simulink model "IEEE_13_BUS_Radial"  (R2021b)
settings: Solver=VariableStepAuto  StartTime=0.0  StopTime=48  RelTol=1e-3
undefined symbols (not defined in the file or in its folder): f611, f632, f633, f634, f645, f646, f650, f652, f671, f675, f680, f684, f692
libraries: simulink x416, slpidlib x13
(part 6 of 7)

== system IEEE_13_BUS_Radial/f645/CONTROLLERS/lPoLC15 ==
  Sum : Sum  Inputs=|++
  base : simulink/Sources/Repeating Sequence Stair  OutValues=f645.PoLC15.l  tsamp=f645.PoLC15.ST  OutMin=[]  OutMax=[]  OutDataTypeStr=double  OutputDataTypeScalingMode=double  OutDataType=fixdt(0,8)  ConRadixGroup=Best Precision: Vector-wise  OutScaling=2^-12
  noise : simulink/Sources/Band-Limited White Noise  Cov=f645.PoLC15.Noise  Ts=f645.PoLC15.NoiseST  seed=f645.PoLC15.NoiseSD
  P : Outport  VectorParamsAs1DForOutWhenUnconnected=off
  wires:
  Sum/1 -> P/1
  noise/1 -> Sum/2
  base/1 -> Sum/1

== system IEEE_13_BUS_Radial/f645/CONTROLLERS/lPoLC16 ==
  cv : Inport
  Sum : Sum  Inputs=|++
  Terminator : Terminator
  base : simulink/Sources/Repeating Sequence Stair  OutValues=f645.PoLC16.l  tsamp=f645.PoLC16.ST  OutMin=[]  OutMax=[]  OutDataTypeStr=double  OutputDataTypeScalingMode=double  OutDataType=fixdt(0,8)  ConRadixGroup=Best Precision: Vector-wise  OutScaling=2^-12
  noise : simulink/Sources/Band-Limited White Noise  Cov=f645.PoLC16.Noise  Ts=f645.PoLC16.NoiseST  seed=f645.PoLC16.NoiseSD
  P : Outport  VectorParamsAs1DForOutWhenUnconnected=off
  wires:
  Sum/1 -> Terminator/1
  noise/1 -> Sum/2
  base/1 -> Sum/1
  cv/1 -> P/1

== system IEEE_13_BUS_Radial/f645/CONTROLLERS/lPoLC2 ==
  Sum : Sum  Inputs=|++
  base : simulink/Sources/Repeating Sequence Stair  OutValues=f645.PoLC2.l  tsamp=f645.PoLC2.ST  OutMin=[]  OutMax=[]  OutDataTypeStr=double  OutputDataTypeScalingMode=double  OutDataType=fixdt(0,8)  ConRadixGroup=Best Precision: Vector-wise  OutScaling=2^-12
  noise : simulink/Sources/Band-Limited White Noise  Cov=f645.PoLC2.Noise  Ts=f645.PoLC2.NoiseST  seed=f645.PoLC2.NoiseSD
  P : Outport  VectorParamsAs1DForOutWhenUnconnected=off
  wires:
  Sum/1 -> P/1
  noise/1 -> Sum/2
  base/1 -> Sum/1

== system IEEE_13_BUS_Radial/f645/CONTROLLERS/lPoLC3 ==
  Sum : Sum  Inputs=|++
  base : simulink/Sources/Repeating Sequence Stair  OutValues=f645.PoLC3.l  tsamp=f645.PoLC3.ST  OutMin=[]  OutMax=[]  OutDataTypeStr=double  OutputDataTypeScalingMode=double  OutDataType=fixdt(0,8)  ConRadixGroup=Best Precision: Vector-wise  OutScaling=2^-12
  noise : simulink/Sources/Band-Limited White Noise  Cov=f645.PoLC3.Noise  Ts=f645.PoLC3.NoiseST  seed=f645.PoLC3.NoiseSD
  P : Outport  VectorParamsAs1DForOutWhenUnconnected=off
  wires:
  Sum/1 -> P/1
  noise/1 -> Sum/2
  base/1 -> Sum/1

== system IEEE_13_BUS_Radial/f645/CONTROLLERS/lPoLC4 ==
  Sum : Sum  Inputs=|++
  base : simulink/Sources/Repeating Sequence Stair  OutValues=f645.PoLC4.l  tsamp=f645.PoLC4.ST  OutMin=[]  OutMax=[]  OutDataTypeStr=double  OutputDataTypeScalingMode=double  OutDataType=fixdt(0,8)  ConRadixGroup=Best Precision: Vector-wise  OutScaling=2^-12
  noise : simulink/Sources/Band-Limited White Noise  Cov=f645.PoLC4.Noise  Ts=f645.PoLC4.NoiseST  seed=f645.PoLC4.NoiseSD
  P : Outport  VectorParamsAs1DForOutWhenUnconnected=off
  wires:
  Sum/1 -> P/1
  noise/1 -> Sum/2
  base/1 -> Sum/1

== system IEEE_13_BUS_Radial/f645/CONTROLLERS/lPoLC5 ==
  Sum : Sum  Inputs=|++
  base : simulink/Sources/Repeating Sequence Stair  OutValues=f645.PoLC5.l  tsamp=f645.PoLC5.ST  OutMin=[]  OutMax=[]  OutDataTypeStr=double  OutputDataTypeScalingMode=double  OutDataType=fixdt(0,8)  ConRadixGroup=Best Precision: Vector-wise  OutScaling=2^-12
  noise : simulink/Sources/Band-Limited White Noise  Cov=f645.PoLC5.Noise  Ts=f645.PoLC5.NoiseST  seed=f645.PoLC5.NoiseSD
  P : Outport  VectorParamsAs1DForOutWhenUnconnected=off
  wires:
  Sum/1 -> P/1
  noise/1 -> Sum/2
  base/1 -> Sum/1

== system IEEE_13_BUS_Radial/f645/CONTROLLERS/lPoLC6 ==
  Sum : Sum  Inputs=|++
  base : simulink/Sources/Repeating Sequence Stair  OutValues=f645.PoLC6.l  tsamp=f645.PoLC6.ST  OutMin=[]  OutMax=[]  OutDataTypeStr=double  OutputDataTypeScalingMode=double  OutDataType=fixdt(0,8)  ConRadixGroup=Best Precision: Vector-wise  OutScaling=2^-12
  noise : simulink/Sources/Band-Limited White Noise  Cov=f645.PoLC6.Noise  Ts=f645.PoLC6.NoiseST  seed=f645.PoLC6.NoiseSD
  P : Outport  VectorParamsAs1DForOutWhenUnconnected=off
  wires:
  Sum/1 -> P/1
  noise/1 -> Sum/2
  base/1 -> Sum/1

== system IEEE_13_BUS_Radial/f645/CONTROLLERS/lPoLC7 ==
  Sum : Sum  Inputs=|++
  base : simulink/Sources/Repeating Sequence Stair  OutValues=f645.PoLC7.l  tsamp=f645.PoLC7.ST  OutMin=[]  OutMax=[]  OutDataTypeStr=double  OutputDataTypeScalingMode=double  OutDataType=fixdt(0,8)  ConRadixGroup=Best Precision: Vector-wise  OutScaling=2^-12
  noise : simulink/Sources/Band-Limited White Noise  Cov=f645.PoLC7.Noise  Ts=f645.PoLC7.NoiseST  seed=f645.PoLC7.NoiseSD
  P : Outport  VectorParamsAs1DForOutWhenUnconnected=off
  wires:
  Sum/1 -> P/1
  noise/1 -> Sum/2
  base/1 -> Sum/1

== system IEEE_13_BUS_Radial/f645/CONTROLLERS/lPoLC8 ==
  Sum : Sum  Inputs=|++
  base : simulink/Sources/Repeating Sequence Stair  OutValues=f645.PoLC8.l  tsamp=f645.PoLC8.ST  OutMin=[]  OutMax=[]  OutDataTypeStr=double  OutputDataTypeScalingMode=double  OutDataType=fixdt(0,8)  ConRadixGroup=Best Precision: Vector-wise  OutScaling=2^-12
  noise : simulink/Sources/Band-Limited White Noise  Cov=f645.PoLC8.Noise  Ts=f645.PoLC8.NoiseST  seed=f645.PoLC8.NoiseSD
  P : Outport  VectorParamsAs1DForOutWhenUnconnected=off
  wires:
  Sum/1 -> P/1
  noise/1 -> Sum/2
  base/1 -> Sum/1

== system IEEE_13_BUS_Radial/f645/CONTROLLERS/lPoLC9 ==
  Sum : Sum  Inputs=|++
  base : simulink/Sources/Repeating Sequence Stair  OutValues=f645.PoLC9.l  tsamp=f645.PoLC9.ST  OutMin=[]  OutMax=[]  OutDataTypeStr=double  OutputDataTypeScalingMode=double  OutDataType=fixdt(0,8)  ConRadixGroup=Best Precision: Vector-wise  OutScaling=2^-12
  noise : simulink/Sources/Band-Limited White Noise  Cov=f645.PoLC9.Noise  Ts=f645.PoLC9.NoiseST  seed=f645.PoLC9.NoiseSD
  P : Outport  VectorParamsAs1DForOutWhenUnconnected=off
  wires:
  Sum/1 -> P/1
  noise/1 -> Sum/2
  base/1 -> Sum/1

== system IEEE_13_BUS_Radial/f645/OPERATIONS GATEWAY/Agent Communications ==
  Enable : EnablePort
  Constant : Constant  Value=0
  Out1 : Outport  VectorParamsAs1DForOutWhenUnconnected=off
  wires:
  Constant/1 -> Out1/1

== system IEEE_13_BUS_Radial/f646/CONTROLLERS/lPoLC1 ==
  Sum : Sum  Inputs=|++
  base : simulink/Sources/Repeating Sequence Stair  OutValues=f646.PoLC1.l  tsamp=f646.PoLC1.ST  OutMin=[]  OutMax=[]  OutDataTypeStr=double  OutputDataTypeScalingMode=double  OutDataType=fixdt(0,8)  ConRadixGroup=Best Precision: Vector-wise  OutScaling=2^-12
  noise : simulink/Sources/Band-Limited White Noise  Cov=f646.PoLC1.Noise  Ts=f646.PoLC1.NoiseST  seed=f646.PoLC1.NoiseSD
  P : Outport  VectorParamsAs1DForOutWhenUnconnected=off
  wires:
  Sum/1 -> P/1
  noise/1 -> Sum/2
  base/1 -> Sum/1

== system IEEE_13_BUS_Radial/f646/CONTROLLERS/lPoLC10 ==
  Sum : Sum  Inputs=|++
  base : simulink/Sources/Repeating Sequence Stair  OutValues=f646.PoLC10.l  tsamp=f646.PoLC10.ST  OutMin=[]  OutMax=[]  OutDataTypeStr=double  OutputDataTypeScalingMode=double  OutDataType=fixdt(0,8)  ConRadixGroup=Best Precision: Vector-wise  OutScaling=2^-12
  noise : simulink/Sources/Band-Limited White Noise  Cov=f646.PoLC10.Noise  Ts=f646.PoLC10.NoiseST  seed=f646.PoLC10.NoiseSD
  P : Outport  VectorParamsAs1DForOutWhenUnconnected=off
  wires:
  Sum/1 -> P/1
  noise/1 -> Sum/2
  base/1 -> Sum/1

== system IEEE_13_BUS_Radial/f646/CONTROLLERS/lPoLC11 ==
  Sum : Sum  Inputs=|++
  base : simulink/Sources/Repeating Sequence Stair  OutValues=f646.PoLC11.l  tsamp=f646.PoLC11.ST  OutMin=[]  OutMax=[]  OutDataTypeStr=double  OutputDataTypeScalingMode=double  OutDataType=fixdt(0,8)  ConRadixGroup=Best Precision: Vector-wise  OutScaling=2^-12
  noise : simulink/Sources/Band-Limited White Noise  Cov=f646.PoLC11.Noise  Ts=f646.PoLC11.NoiseST  seed=f646.PoLC11.NoiseSD
  P : Outport  VectorParamsAs1DForOutWhenUnconnected=off
  wires:
  Sum/1 -> P/1
  noise/1 -> Sum/2
  base/1 -> Sum/1

== system IEEE_13_BUS_Radial/f646/CONTROLLERS/lPoLC12 ==
  Sum : Sum  Inputs=|++
  base : simulink/Sources/Repeating Sequence Stair  OutValues=f646.PoLC12.l  tsamp=f646.PoLC12.ST  OutMin=[]  OutMax=[]  OutDataTypeStr=double  OutputDataTypeScalingMode=double  OutDataType=fixdt(0,8)  ConRadixGroup=Best Precision: Vector-wise  OutScaling=2^-12
  noise : simulink/Sources/Band-Limited White Noise  Cov=f646.PoLC12.Noise  Ts=f646.PoLC12.NoiseST  seed=f646.PoLC12.NoiseSD
  P : Outport  VectorParamsAs1DForOutWhenUnconnected=off
  wires:
  Sum/1 -> P/1
  noise/1 -> Sum/2
  base/1 -> Sum/1

== system IEEE_13_BUS_Radial/f646/CONTROLLERS/lPoLC13 ==
  Sum : Sum  Inputs=|++
  base : simulink/Sources/Repeating Sequence Stair  OutValues=f646.PoLC13.l  tsamp=f646.PoLC13.ST  OutMin=[]  OutMax=[]  OutDataTypeStr=double  OutputDataTypeScalingMode=double  OutDataType=fixdt(0,8)  ConRadixGroup=Best Precision: Vector-wise  OutScaling=2^-12
  noise : simulink/Sources/Band-Limited White Noise  Cov=f646.PoLC13.Noise  Ts=f646.PoLC13.NoiseST  seed=f646.PoLC13.NoiseSD
  P : Outport  VectorParamsAs1DForOutWhenUnconnected=off
  wires:
  Sum/1 -> P/1
  noise/1 -> Sum/2
  base/1 -> Sum/1

== system IEEE_13_BUS_Radial/f646/CONTROLLERS/lPoLC14 ==
  Sum : Sum  Inputs=|++
  base : simulink/Sources/Repeating Sequence Stair  OutValues=f646.PoLC14.l  tsamp=f646.PoLC14.ST  OutMin=[]  OutMax=[]  OutDataTypeStr=double  OutputDataTypeScalingMode=double  OutDataType=fixdt(0,8)  ConRadixGroup=Best Precision: Vector-wise  OutScaling=2^-12
  noise : simulink/Sources/Band-Limited White Noise  Cov=f646.PoLC14.Noise  Ts=f646.PoLC14.NoiseST  seed=f646.PoLC14.NoiseSD
  P : Outport  VectorParamsAs1DForOutWhenUnconnected=off
  wires:
  Sum/1 -> P/1
  noise/1 -> Sum/2
  base/1 -> Sum/1

== system IEEE_13_BUS_Radial/f646/CONTROLLERS/lPoLC15 ==
  Sum : Sum  Inputs=|++
  base : simulink/Sources/Repeating Sequence Stair  OutValues=f646.PoLC15.l  tsamp=f646.PoLC15.ST  OutMin=[]  OutMax=[]  OutDataTypeStr=double  OutputDataTypeScalingMode=double  OutDataType=fixdt(0,8)  ConRadixGroup=Best Precision: Vector-wise  OutScaling=2^-12
  noise : simulink/Sources/Band-Limited White Noise  Cov=f646.PoLC15.Noise  Ts=f646.PoLC15.NoiseST  seed=f646.PoLC15.NoiseSD
  P : Outport  VectorParamsAs1DForOutWhenUnconnected=off
  wires:
  Sum/1 -> P/1
  noise/1 -> Sum/2
  base/1 -> Sum/1

== system IEEE_13_BUS_Radial/f646/CONTROLLERS/lPoLC16 ==
  cv : Inport
  Sum : Sum  Inputs=|++
  Terminator : Terminator
  base : simulink/Sources/Repeating Sequence Stair  OutValues=f646.PoLC16.l  tsamp=f646.PoLC16.ST  OutMin=[]  OutMax=[]  OutDataTypeStr=double  OutputDataTypeScalingMode=double  OutDataType=fixdt(0,8)  ConRadixGroup=Best Precision: Vector-wise  OutScaling=2^-12
  noise : simulink/Sources/Band-Limited White Noise  Cov=f646.PoLC16.Noise  Ts=f646.PoLC16.NoiseST  seed=f646.PoLC16.NoiseSD
  P : Outport  VectorParamsAs1DForOutWhenUnconnected=off
  wires:
  Sum/1 -> Terminator/1
  noise/1 -> Sum/2
  base/1 -> Sum/1
  cv/1 -> P/1

== system IEEE_13_BUS_Radial/f646/CONTROLLERS/lPoLC2 ==
  Sum : Sum  Inputs=|++
  base : simulink/Sources/Repeating Sequence Stair  OutValues=f646.PoLC2.l  tsamp=f646.PoLC2.ST  OutMin=[]  OutMax=[]  OutDataTypeStr=double  OutputDataTypeScalingMode=double  OutDataType=fixdt(0,8)  ConRadixGroup=Best Precision: Vector-wise  OutScaling=2^-12
  noise : simulink/Sources/Band-Limited White Noise  Cov=f646.PoLC2.Noise  Ts=f646.PoLC2.NoiseST  seed=f646.PoLC2.NoiseSD
  P : Outport  VectorParamsAs1DForOutWhenUnconnected=off
  wires:
  Sum/1 -> P/1
  noise/1 -> Sum/2
  base/1 -> Sum/1

== system IEEE_13_BUS_Radial/f646/CONTROLLERS/lPoLC3 ==
  Sum : Sum  Inputs=|++
  base : simulink/Sources/Repeating Sequence Stair  OutValues=f646.PoLC3.l  tsamp=f646.PoLC3.ST  OutMin=[]  OutMax=[]  OutDataTypeStr=double  OutputDataTypeScalingMode=double  OutDataType=fixdt(0,8)  ConRadixGroup=Best Precision: Vector-wise  OutScaling=2^-12
  noise : simulink/Sources/Band-Limited White Noise  Cov=f646.PoLC3.Noise  Ts=f646.PoLC3.NoiseST  seed=f646.PoLC3.NoiseSD
  P : Outport  VectorParamsAs1DForOutWhenUnconnected=off
  wires:
  Sum/1 -> P/1
  noise/1 -> Sum/2
  base/1 -> Sum/1

== system IEEE_13_BUS_Radial/f646/CONTROLLERS/lPoLC4 ==
  Sum : Sum  Inputs=|++
  base : simulink/Sources/Repeating Sequence Stair  OutValues=f646.PoLC4.l  tsamp=f646.PoLC4.ST  OutMin=[]  OutMax=[]  OutDataTypeStr=double  OutputDataTypeScalingMode=double  OutDataType=fixdt(0,8)  ConRadixGroup=Best Precision: Vector-wise  OutScaling=2^-12
  noise : simulink/Sources/Band-Limited White Noise  Cov=f646.PoLC4.Noise  Ts=f646.PoLC4.NoiseST  seed=f646.PoLC4.NoiseSD
  P : Outport  VectorParamsAs1DForOutWhenUnconnected=off
  wires:
  Sum/1 -> P/1
  noise/1 -> Sum/2
  base/1 -> Sum/1

== system IEEE_13_BUS_Radial/f646/CONTROLLERS/lPoLC5 ==
  Sum : Sum  Inputs=|++
  base : simulink/Sources/Repeating Sequence Stair  OutValues=f646.PoLC5.l  tsamp=f646.PoLC5.ST  OutMin=[]  OutMax=[]  OutDataTypeStr=double  OutputDataTypeScalingMode=double  OutDataType=fixdt(0,8)  ConRadixGroup=Best Precision: Vector-wise  OutScaling=2^-12
  noise : simulink/Sources/Band-Limited White Noise  Cov=f646.PoLC5.Noise  Ts=f646.PoLC5.NoiseST  seed=f646.PoLC5.NoiseSD
  P : Outport  VectorParamsAs1DForOutWhenUnconnected=off
  wires:
  Sum/1 -> P/1
  noise/1 -> Sum/2
  base/1 -> Sum/1

== system IEEE_13_BUS_Radial/f646/CONTROLLERS/lPoLC6 ==
  Sum : Sum  Inputs=|++
  base : simulink/Sources/Repeating Sequence Stair  OutValues=f646.PoLC6.l  tsamp=f646.PoLC6.ST  OutMin=[]  OutMax=[]  OutDataTypeStr=double  OutputDataTypeScalingMode=double  OutDataType=fixdt(0,8)  ConRadixGroup=Best Precision: Vector-wise  OutScaling=2^-12
  noise : simulink/Sources/Band-Limited White Noise  Cov=f646.PoLC6.Noise  Ts=f646.PoLC6.NoiseST  seed=f646.PoLC6.NoiseSD
  P : Outport  VectorParamsAs1DForOutWhenUnconnected=off
  wires:
  Sum/1 -> P/1
  noise/1 -> Sum/2
  base/1 -> Sum/1

== system IEEE_13_BUS_Radial/f646/CONTROLLERS/lPoLC7 ==
  Sum : Sum  Inputs=|++
  base : simulink/Sources/Repeating Sequence Stair  OutValues=f646.PoLC7.l  tsamp=f646.PoLC7.ST  OutMin=[]  OutMax=[]  OutDataTypeStr=double  OutputDataTypeScalingMode=double  OutDataType=fixdt(0,8)  ConRadixGroup=Best Precision: Vector-wise  OutScaling=2^-12
  noise : simulink/Sources/Band-Limited White Noise  Cov=f646.PoLC7.Noise  Ts=f646.PoLC7.NoiseST  seed=f646.PoLC7.NoiseSD
  P : Outport  VectorParamsAs1DForOutWhenUnconnected=off
  wires:
  Sum/1 -> P/1
  noise/1 -> Sum/2
  base/1 -> Sum/1

== system IEEE_13_BUS_Radial/f646/CONTROLLERS/lPoLC8 ==
  Sum : Sum  Inputs=|++
  base : simulink/Sources/Repeating Sequence Stair  OutValues=f646.PoLC8.l  tsamp=f646.PoLC8.ST  OutMin=[]  OutMax=[]  OutDataTypeStr=double  OutputDataTypeScalingMode=double  OutDataType=fixdt(0,8)  ConRadixGroup=Best Precision: Vector-wise  OutScaling=2^-12
  noise : simulink/Sources/Band-Limited White Noise  Cov=f646.PoLC8.Noise  Ts=f646.PoLC8.NoiseST  seed=f646.PoLC8.NoiseSD
  P : Outport  VectorParamsAs1DForOutWhenUnconnected=off
  wires:
  Sum/1 -> P/1
  noise/1 -> Sum/2
  base/1 -> Sum/1

== system IEEE_13_BUS_Radial/f646/CONTROLLERS/lPoLC9 ==
  Sum : Sum  Inputs=|++
  base : simulink/Sources/Repeating Sequence Stair  OutValues=f646.PoLC9.l  tsamp=f646.PoLC9.ST  OutMin=[]  OutMax=[]  OutDataTypeStr=double  OutputDataTypeScalingMode=double  OutDataType=fixdt(0,8)  ConRadixGroup=Best Precision: Vector-wise  OutScaling=2^-12
  noise : simulink/Sources/Band-Limited White Noise  Cov=f646.PoLC9.Noise  Ts=f646.PoLC9.NoiseST  seed=f646.PoLC9.NoiseSD
  P : Outport  VectorParamsAs1DForOutWhenUnconnected=off
  wires:
  Sum/1 -> P/1
  noise/1 -> Sum/2
  base/1 -> Sum/1

== system IEEE_13_BUS_Radial/f646/OPERATIONS GATEWAY/Agent Communications ==
  Enable : EnablePort
  Constant : Constant  Value=0
  Out1 : Outport  VectorParamsAs1DForOutWhenUnconnected=off
  wires:
  Constant/1 -> Out1/1

== system IEEE_13_BUS_Radial/f650/CONTROLLERS/lPoLC1 ==
  Sum : Sum  Inputs=|++
  base : simulink/Sources/Repeating Sequence Stair  OutValues=f650.PoLC1.l  tsamp=f650.PoLC1.ST  OutMin=[]  OutMax=[]  OutDataTypeStr=double  OutputDataTypeScalingMode=double  OutDataType=fixdt(0,8)  ConRadixGroup=Best Precision: Vector-wise  OutScaling=2^-12
  noise : simulink/Sources/Band-Limited White Noise  Cov=f650.PoLC1.Noise  Ts=f650.PoLC1.NoiseST  seed=f650.PoLC1.NoiseSD
  P : Outport  VectorParamsAs1DForOutWhenUnconnected=off
  wires:
  Sum/1 -> P/1
  noise/1 -> Sum/2
  base/1 -> Sum/1

== system IEEE_13_BUS_Radial/f650/CONTROLLERS/lPoLC10 ==
  Sum : Sum  Inputs=|++
  base : simulink/Sources/Repeating Sequence Stair  OutValues=f650.PoLC10.l  tsamp=f650.PoLC10.ST  OutMin=[]  OutMax=[]  OutDataTypeStr=double  OutputDataTypeScalingMode=double  OutDataType=fixdt(0,8)  ConRadixGroup=Best Precision: Vector-wise  OutScaling=2^-12
  noise : simulink/Sources/Band-Limited White Noise  Cov=f650.PoLC10.Noise  Ts=f650.PoLC10.NoiseST  seed=f650.PoLC10.NoiseSD
  P : Outport  VectorParamsAs1DForOutWhenUnconnected=off
  wires:
  Sum/1 -> P/1
  noise/1 -> Sum/2
  base/1 -> Sum/1

== system IEEE_13_BUS_Radial/f650/CONTROLLERS/lPoLC11 ==
  Sum : Sum  Inputs=|++
  base : simulink/Sources/Repeating Sequence Stair  OutValues=f650.PoLC11.l  tsamp=f650.PoLC11.ST  OutMin=[]  OutMax=[]  OutDataTypeStr=double  OutputDataTypeScalingMode=double  OutDataType=fixdt(0,8)  ConRadixGroup=Best Precision: Vector-wise  OutScaling=2^-12
  noise : simulink/Sources/Band-Limited White Noise  Cov=f650.PoLC11.Noise  Ts=f650.PoLC11.NoiseST  seed=f650.PoLC11.NoiseSD
  P : Outport  VectorParamsAs1DForOutWhenUnconnected=off
  wires:
  Sum/1 -> P/1
  noise/1 -> Sum/2
  base/1 -> Sum/1

== system IEEE_13_BUS_Radial/f650/CONTROLLERS/lPoLC12 ==
  Sum : Sum  Inputs=|++
  base : simulink/Sources/Repeating Sequence Stair  OutValues=f650.PoLC12.l  tsamp=f650.PoLC12.ST  OutMin=[]  OutMax=[]  OutDataTypeStr=double  OutputDataTypeScalingMode=double  OutDataType=fixdt(0,8)  ConRadixGroup=Best Precision: Vector-wise  OutScaling=2^-12
  noise : simulink/Sources/Band-Limited White Noise  Cov=f650.PoLC12.Noise  Ts=f650.PoLC12.NoiseST  seed=f650.PoLC12.NoiseSD
  P : Outport  VectorParamsAs1DForOutWhenUnconnected=off
  wires:
  Sum/1 -> P/1
  noise/1 -> Sum/2
  base/1 -> Sum/1

== system IEEE_13_BUS_Radial/f650/CONTROLLERS/lPoLC13 ==
  Sum : Sum  Inputs=|++
  base : simulink/Sources/Repeating Sequence Stair  OutValues=f650.PoLC13.l  tsamp=f650.PoLC13.ST  OutMin=[]  OutMax=[]  OutDataTypeStr=double  OutputDataTypeScalingMode=double  OutDataType=fixdt(0,8)  ConRadixGroup=Best Precision: Vector-wise  OutScaling=2^-12
  noise : simulink/Sources/Band-Limited White Noise  Cov=f650.PoLC13.Noise  Ts=f650.PoLC13.NoiseST  seed=f650.PoLC13.NoiseSD
  P : Outport  VectorParamsAs1DForOutWhenUnconnected=off
  wires:
  Sum/1 -> P/1
  noise/1 -> Sum/2
  base/1 -> Sum/1

== system IEEE_13_BUS_Radial/f650/CONTROLLERS/lPoLC14 ==
  Sum : Sum  Inputs=|++
  base : simulink/Sources/Repeating Sequence Stair  OutValues=f650.PoLC14.l  tsamp=f650.PoLC14.ST  OutMin=[]  OutMax=[]  OutDataTypeStr=double  OutputDataTypeScalingMode=double  OutDataType=fixdt(0,8)  ConRadixGroup=Best Precision: Vector-wise  OutScaling=2^-12
  noise : simulink/Sources/Band-Limited White Noise  Cov=f650.PoLC14.Noise  Ts=f650.PoLC14.NoiseST  seed=f650.PoLC14.NoiseSD
  P : Outport  VectorParamsAs1DForOutWhenUnconnected=off
  wires:
  Sum/1 -> P/1
  noise/1 -> Sum/2
  base/1 -> Sum/1

== system IEEE_13_BUS_Radial/f650/CONTROLLERS/lPoLC15 ==
  Sum : Sum  Inputs=|++
  base : simulink/Sources/Repeating Sequence Stair  OutValues=f650.PoLC15.l  tsamp=f650.PoLC15.ST  OutMin=[]  OutMax=[]  OutDataTypeStr=double  OutputDataTypeScalingMode=double  OutDataType=fixdt(0,8)  ConRadixGroup=Best Precision: Vector-wise  OutScaling=2^-12
  noise : simulink/Sources/Band-Limited White Noise  Cov=f650.PoLC15.Noise  Ts=f650.PoLC15.NoiseST  seed=f650.PoLC15.NoiseSD
  P : Outport  VectorParamsAs1DForOutWhenUnconnected=off
  wires:
  Sum/1 -> P/1
  noise/1 -> Sum/2
  base/1 -> Sum/1

== system IEEE_13_BUS_Radial/f650/CONTROLLERS/lPoLC16 ==
  cv : Inport
  Sum : Sum  Inputs=|++
  Terminator : Terminator
  base : simulink/Sources/Repeating Sequence Stair  OutValues=f650.PoLC16.l  tsamp=f650.PoLC16.ST  OutMin=[]  OutMax=[]  OutDataTypeStr=double  OutputDataTypeScalingMode=double  OutDataType=fixdt(0,8)  ConRadixGroup=Best Precision: Vector-wise  OutScaling=2^-12
  noise : simulink/Sources/Band-Limited White Noise  Cov=f650.PoLC16.Noise  Ts=f650.PoLC16.NoiseST  seed=f650.PoLC16.NoiseSD
  P : Outport  VectorParamsAs1DForOutWhenUnconnected=off
  wires:
  Sum/1 -> Terminator/1
  noise/1 -> Sum/2
  base/1 -> Sum/1
  cv/1 -> P/1

== system IEEE_13_BUS_Radial/f650/CONTROLLERS/lPoLC2 ==
  Sum : Sum  Inputs=|++
  base : simulink/Sources/Repeating Sequence Stair  OutValues=f650.PoLC2.l  tsamp=f650.PoLC2.ST  OutMin=[]  OutMax=[]  OutDataTypeStr=double  OutputDataTypeScalingMode=double  OutDataType=fixdt(0,8)  ConRadixGroup=Best Precision: Vector-wise  OutScaling=2^-12
  noise : simulink/Sources/Band-Limited White Noise  Cov=f650.PoLC2.Noise  Ts=f650.PoLC2.NoiseST  seed=f650.PoLC2.NoiseSD
  P : Outport  VectorParamsAs1DForOutWhenUnconnected=off
  wires:
  Sum/1 -> P/1
  noise/1 -> Sum/2
  base/1 -> Sum/1

== system IEEE_13_BUS_Radial/f650/CONTROLLERS/lPoLC3 ==
  Sum : Sum  Inputs=|++
  base : simulink/Sources/Repeating Sequence Stair  OutValues=f650.PoLC3.l  tsamp=f650.PoLC3.ST  OutMin=[]  OutMax=[]  OutDataTypeStr=double  OutputDataTypeScalingMode=double  OutDataType=fixdt(0,8)  ConRadixGroup=Best Precision: Vector-wise  OutScaling=2^-12
  noise : simulink/Sources/Band-Limited White Noise  Cov=f650.PoLC3.Noise  Ts=f650.PoLC3.NoiseST  seed=f650.PoLC3.NoiseSD
  P : Outport  VectorParamsAs1DForOutWhenUnconnected=off
  wires:
  Sum/1 -> P/1
  noise/1 -> Sum/2
  base/1 -> Sum/1

== system IEEE_13_BUS_Radial/f650/CONTROLLERS/lPoLC4 ==
  Sum : Sum  Inputs=|++
  base : simulink/Sources/Repeating Sequence Stair  OutValues=f650.PoLC4.l  tsamp=f650.PoLC4.ST  OutMin=[]  OutMax=[]  OutDataTypeStr=double  OutputDataTypeScalingMode=double  OutDataType=fixdt(0,8)  ConRadixGroup=Best Precision: Vector-wise  OutScaling=2^-12
  noise : simulink/Sources/Band-Limited White Noise  Cov=f650.PoLC4.Noise  Ts=f650.PoLC4.NoiseST  seed=f650.PoLC4.NoiseSD
  P : Outport  VectorParamsAs1DForOutWhenUnconnected=off
  wires:
  Sum/1 -> P/1
  noise/1 -> Sum/2
  base/1 -> Sum/1

== system IEEE_13_BUS_Radial/f650/CONTROLLERS/lPoLC5 ==
  Sum : Sum  Inputs=|++
  base : simulink/Sources/Repeating Sequence Stair  OutValues=f650.PoLC5.l  tsamp=f650.PoLC5.ST  OutMin=[]  OutMax=[]  OutDataTypeStr=double  OutputDataTypeScalingMode=double  OutDataType=fixdt(0,8)  ConRadixGroup=Best Precision: Vector-wise  OutScaling=2^-12
  noise : simulink/Sources/Band-Limited White Noise  Cov=f650.PoLC5.Noise  Ts=f650.PoLC5.NoiseST  seed=f650.PoLC5.NoiseSD
  P : Outport  VectorParamsAs1DForOutWhenUnconnected=off
  wires:
  Sum/1 -> P/1
  noise/1 -> Sum/2
  base/1 -> Sum/1

== system IEEE_13_BUS_Radial/f650/CONTROLLERS/lPoLC6 ==
  Sum : Sum  Inputs=|++
  base : simulink/Sources/Repeating Sequence Stair  OutValues=f650.PoLC6.l  tsamp=f650.PoLC6.ST  OutMin=[]  OutMax=[]  OutDataTypeStr=double  OutputDataTypeScalingMode=double  OutDataType=fixdt(0,8)  ConRadixGroup=Best Precision: Vector-wise  OutScaling=2^-12
  noise : simulink/Sources/Band-Limited White Noise  Cov=f650.PoLC6.Noise  Ts=f650.PoLC6.NoiseST  seed=f650.PoLC6.NoiseSD
  P : Outport  VectorParamsAs1DForOutWhenUnconnected=off
  wires:
  Sum/1 -> P/1
  noise/1 -> Sum/2
  base/1 -> Sum/1

== system IEEE_13_BUS_Radial/f650/CONTROLLERS/lPoLC7 ==
  Sum : Sum  Inputs=|++
  base : simulink/Sources/Repeating Sequence Stair  OutValues=f650.PoLC7.l  tsamp=f650.PoLC7.ST  OutMin=[]  OutMax=[]  OutDataTypeStr=double  OutputDataTypeScalingMode=double  OutDataType=fixdt(0,8)  ConRadixGroup=Best Precision: Vector-wise  OutScaling=2^-12
  noise : simulink/Sources/Band-Limited White Noise  Cov=f650.PoLC7.Noise  Ts=f650.PoLC7.NoiseST  seed=f650.PoLC7.NoiseSD
  P : Outport  VectorParamsAs1DForOutWhenUnconnected=off
  wires:
  Sum/1 -> P/1
  noise/1 -> Sum/2
  base/1 -> Sum/1

== system IEEE_13_BUS_Radial/f650/CONTROLLERS/lPoLC8 ==
  Sum : Sum  Inputs=|++
  base : simulink/Sources/Repeating Sequence Stair  OutValues=f650.PoLC8.l  tsamp=f650.PoLC8.ST  OutMin=[]  OutMax=[]  OutDataTypeStr=double  OutputDataTypeScalingMode=double  OutDataType=fixdt(0,8)  ConRadixGroup=Best Precision: Vector-wise  OutScaling=2^-12
  noise : simulink/Sources/Band-Limited White Noise  Cov=f650.PoLC8.Noise  Ts=f650.PoLC8.NoiseST  seed=f650.PoLC8.NoiseSD
  P : Outport  VectorParamsAs1DForOutWhenUnconnected=off
  wires:
  Sum/1 -> P/1
  noise/1 -> Sum/2
  base/1 -> Sum/1

== system IEEE_13_BUS_Radial/f650/CONTROLLERS/lPoLC9 ==
  Sum : Sum  Inputs=|++
  base : simulink/Sources/Repeating Sequence Stair  OutValues=f650.PoLC9.l  tsamp=f650.PoLC9.ST  OutMin=[]  OutMax=[]  OutDataTypeStr=double  OutputDataTypeScalingMode=double  OutDataType=fixdt(0,8)  ConRadixGroup=Best Precision: Vector-wise  OutScaling=2^-12
  noise : simulink/Sources/Band-Limited White Noise  Cov=f650.PoLC9.Noise  Ts=f650.PoLC9.NoiseST  seed=f650.PoLC9.NoiseSD
  P : Outport  VectorParamsAs1DForOutWhenUnconnected=off
  wires:
  Sum/1 -> P/1
  noise/1 -> Sum/2
  base/1 -> Sum/1

== system IEEE_13_BUS_Radial/f650/OPERATIONS GATEWAY/Agent Communications ==
  Enable : EnablePort
  Constant : Constant  Value=0
  Out1 : Outport  VectorParamsAs1DForOutWhenUnconnected=off
  wires:
  Constant/1 -> Out1/1

== system IEEE_13_BUS_Radial/f652/CONTROLLERS/lPoLC1 ==
  Sum : Sum  Inputs=|++
  base : simulink/Sources/Repeating Sequence Stair  OutValues=f652.PoLC1.l  tsamp=f652.PoLC1.ST  OutMin=[]  OutMax=[]  OutDataTypeStr=double  OutputDataTypeScalingMode=double  OutDataType=fixdt(0,8)  ConRadixGroup=Best Precision: Vector-wise  OutScaling=2^-12
  noise : simulink/Sources/Band-Limited White Noise  Cov=f652.PoLC1.Noise  Ts=f652.PoLC1.NoiseST  seed=f652.PoLC1.NoiseSD
  P : Outport  VectorParamsAs1DForOutWhenUnconnected=off
  wires:
  Sum/1 -> P/1
  noise/1 -> Sum/2
  base/1 -> Sum/1

== system IEEE_13_BUS_Radial/f652/CONTROLLERS/lPoLC10 ==
  Sum : Sum  Inputs=|++
  base : simulink/Sources/Repeating Sequence Stair  OutValues=f652.PoLC10.l  tsamp=f652.PoLC10.ST  OutMin=[]  OutMax=[]  OutDataTypeStr=double  OutputDataTypeScalingMode=double  OutDataType=fixdt(0,8)  ConRadixGroup=Best Precision: Vector-wise  OutScaling=2^-12
  noise : simulink/Sources/Band-Limited White Noise  Cov=f652.PoLC10.Noise  Ts=f652.PoLC10.NoiseST  seed=f652.PoLC10.NoiseSD
  P : Outport  VectorParamsAs1DForOutWhenUnconnected=off
  wires:
  Sum/1 -> P/1
  noise/1 -> Sum/2
  base/1 -> Sum/1

== system IEEE_13_BUS_Radial/f652/CONTROLLERS/lPoLC11 ==
  Sum : Sum  Inputs=|++
  base : simulink/Sources/Repeating Sequence Stair  OutValues=f652.PoLC11.l  tsamp=f652.PoLC11.ST  OutMin=[]  OutMax=[]  OutDataTypeStr=double  OutputDataTypeScalingMode=double  OutDataType=fixdt(0,8)  ConRadixGroup=Best Precision: Vector-wise  OutScaling=2^-12
  noise : simulink/Sources/Band-Limited White Noise  Cov=f652.PoLC11.Noise  Ts=f652.PoLC11.NoiseST  seed=f652.PoLC11.NoiseSD
  P : Outport  VectorParamsAs1DForOutWhenUnconnected=off
  wires:
  Sum/1 -> P/1
  noise/1 -> Sum/2
  base/1 -> Sum/1

== system IEEE_13_BUS_Radial/f652/CONTROLLERS/lPoLC12 ==
  Sum : Sum  Inputs=|++
  base : simulink/Sources/Repeating Sequence Stair  OutValues=f652.PoLC12.l  tsamp=f652.PoLC12.ST  OutMin=[]  OutMax=[]  OutDataTypeStr=double  OutputDataTypeScalingMode=double  OutDataType=fixdt(0,8)  ConRadixGroup=Best Precision: Vector-wise  OutScaling=2^-12
  noise : simulink/Sources/Band-Limited White Noise  Cov=f652.PoLC12.Noise  Ts=f652.PoLC12.NoiseST  seed=f652.PoLC12.NoiseSD
  P : Outport  VectorParamsAs1DForOutWhenUnconnected=off
  wires:
  Sum/1 -> P/1
  noise/1 -> Sum/2
  base/1 -> Sum/1

== system IEEE_13_BUS_Radial/f652/CONTROLLERS/lPoLC13 ==
  Sum : Sum  Inputs=|++
  base : simulink/Sources/Repeating Sequence Stair  OutValues=f652.PoLC13.l  tsamp=f652.PoLC13.ST  OutMin=[]  OutMax=[]  OutDataTypeStr=double  OutputDataTypeScalingMode=double  OutDataType=fixdt(0,8)  ConRadixGroup=Best Precision: Vector-wise  OutScaling=2^-12
  noise : simulink/Sources/Band-Limited White Noise  Cov=f652.PoLC13.Noise  Ts=f652.PoLC13.NoiseST  seed=f652.PoLC13.NoiseSD
  P : Outport  VectorParamsAs1DForOutWhenUnconnected=off
  wires:
  Sum/1 -> P/1
  noise/1 -> Sum/2
  base/1 -> Sum/1

== system IEEE_13_BUS_Radial/f652/CONTROLLERS/lPoLC14 ==
  Sum : Sum  Inputs=|++
  base : simulink/Sources/Repeating Sequence Stair  OutValues=f652.PoLC14.l  tsamp=f652.PoLC14.ST  OutMin=[]  OutMax=[]  OutDataTypeStr=double  OutputDataTypeScalingMode=double  OutDataType=fixdt(0,8)  ConRadixGroup=Best Precision: Vector-wise  OutScaling=2^-12
  noise : simulink/Sources/Band-Limited White Noise  Cov=f652.PoLC14.Noise  Ts=f652.PoLC14.NoiseST  seed=f652.PoLC14.NoiseSD
  P : Outport  VectorParamsAs1DForOutWhenUnconnected=off
  wires:
  Sum/1 -> P/1
  noise/1 -> Sum/2
  base/1 -> Sum/1

== system IEEE_13_BUS_Radial/f652/CONTROLLERS/lPoLC15 ==
  Sum : Sum  Inputs=|++
  base : simulink/Sources/Repeating Sequence Stair  OutValues=f652.PoLC15.l  tsamp=f652.PoLC15.ST  OutMin=[]  OutMax=[]  OutDataTypeStr=double  OutputDataTypeScalingMode=double  OutDataType=fixdt(0,8)  ConRadixGroup=Best Precision: Vector-wise  OutScaling=2^-12
  noise : simulink/Sources/Band-Limited White Noise  Cov=f652.PoLC15.Noise  Ts=f652.PoLC15.NoiseST  seed=f652.PoLC15.NoiseSD
  P : Outport  VectorParamsAs1DForOutWhenUnconnected=off
  wires:
  Sum/1 -> P/1
  noise/1 -> Sum/2
  base/1 -> Sum/1

== system IEEE_13_BUS_Radial/f652/CONTROLLERS/lPoLC16 ==
  cv : Inport
  Sum : Sum  Inputs=|++
  Terminator : Terminator
  base : simulink/Sources/Repeating Sequence Stair  OutValues=f652.PoLC16.l  tsamp=f652.PoLC16.ST  OutMin=[]  OutMax=[]  OutDataTypeStr=double  OutputDataTypeScalingMode=double  OutDataType=fixdt(0,8)  ConRadixGroup=Best Precision: Vector-wise  OutScaling=2^-12
  noise : simulink/Sources/Band-Limited White Noise  Cov=f652.PoLC16.Noise  Ts=f652.PoLC16.NoiseST  seed=f652.PoLC16.NoiseSD
  P : Outport  VectorParamsAs1DForOutWhenUnconnected=off
  wires:
  Sum/1 -> Terminator/1
  noise/1 -> Sum/2
  base/1 -> Sum/1
  cv/1 -> P/1

== system IEEE_13_BUS_Radial/f652/CONTROLLERS/lPoLC2 ==
  Sum : Sum  Inputs=|++
  base : simulink/Sources/Repeating Sequence Stair  OutValues=f652.PoLC2.l  tsamp=f652.PoLC2.ST  OutMin=[]  OutMax=[]  OutDataTypeStr=double  OutputDataTypeScalingMode=double  OutDataType=fixdt(0,8)  ConRadixGroup=Best Precision: Vector-wise  OutScaling=2^-12
  noise : simulink/Sources/Band-Limited White Noise  Cov=f652.PoLC2.Noise  Ts=f652.PoLC2.NoiseST  seed=f652.PoLC2.NoiseSD
  P : Outport  VectorParamsAs1DForOutWhenUnconnected=off
  wires:
  Sum/1 -> P/1
  noise/1 -> Sum/2
  base/1 -> Sum/1

== system IEEE_13_BUS_Radial/f652/CONTROLLERS/lPoLC3 ==
  Sum : Sum  Inputs=|++
  base : simulink/Sources/Repeating Sequence Stair  OutValues=f652.PoLC3.l  tsamp=f652.PoLC3.ST  OutMin=[]  OutMax=[]  OutDataTypeStr=double  OutputDataTypeScalingMode=double  OutDataType=fixdt(0,8)  ConRadixGroup=Best Precision: Vector-wise  OutScaling=2^-12
  noise : simulink/Sources/Band-Limited White Noise  Cov=f652.PoLC3.Noise  Ts=f652.PoLC3.NoiseST  seed=f652.PoLC3.NoiseSD
  P : Outport  VectorParamsAs1DForOutWhenUnconnected=off
  wires:
  Sum/1 -> P/1
  noise/1 -> Sum/2
  base/1 -> Sum/1

== system IEEE_13_BUS_Radial/f652/CONTROLLERS/lPoLC4 ==
  Sum : Sum  Inputs=|++
  base : simulink/Sources/Repeating Sequence Stair  OutValues=f652.PoLC4.l  tsamp=f652.PoLC4.ST  OutMin=[]  OutMax=[]  OutDataTypeStr=double  OutputDataTypeScalingMode=double  OutDataType=fixdt(0,8)  ConRadixGroup=Best Precision: Vector-wise  OutScaling=2^-12
  noise : simulink/Sources/Band-Limited White Noise  Cov=f652.PoLC4.Noise  Ts=f652.PoLC4.NoiseST  seed=f652.PoLC4.NoiseSD
  P : Outport  VectorParamsAs1DForOutWhenUnconnected=off
  wires:
  Sum/1 -> P/1
  noise/1 -> Sum/2
  base/1 -> Sum/1

== system IEEE_13_BUS_Radial/f652/CONTROLLERS/lPoLC5 ==
  Sum : Sum  Inputs=|++
  base : simulink/Sources/Repeating Sequence Stair  OutValues=f652.PoLC5.l  tsamp=f652.PoLC5.ST  OutMin=[]  OutMax=[]  OutDataTypeStr=double  OutputDataTypeScalingMode=double  OutDataType=fixdt(0,8)  ConRadixGroup=Best Precision: Vector-wise  OutScaling=2^-12
  noise : simulink/Sources/Band-Limited White Noise  Cov=f652.PoLC5.Noise  Ts=f652.PoLC5.NoiseST  seed=f652.PoLC5.NoiseSD
  P : Outport  VectorParamsAs1DForOutWhenUnconnected=off
  wires:
  Sum/1 -> P/1
  noise/1 -> Sum/2
  base/1 -> Sum/1

== system IEEE_13_BUS_Radial/f652/CONTROLLERS/lPoLC6 ==
  Sum : Sum  Inputs=|++
  base : simulink/Sources/Repeating Sequence Stair  OutValues=f652.PoLC6.l  tsamp=f652.PoLC6.ST  OutMin=[]  OutMax=[]  OutDataTypeStr=double  OutputDataTypeScalingMode=double  OutDataType=fixdt(0,8)  ConRadixGroup=Best Precision: Vector-wise  OutScaling=2^-12
  noise : simulink/Sources/Band-Limited White Noise  Cov=f652.PoLC6.Noise  Ts=f652.PoLC6.NoiseST  seed=f652.PoLC6.NoiseSD
  P : Outport  VectorParamsAs1DForOutWhenUnconnected=off
  wires:
  Sum/1 -> P/1
  noise/1 -> Sum/2
  base/1 -> Sum/1

== system IEEE_13_BUS_Radial/f652/CONTROLLERS/lPoLC7 ==
  Sum : Sum  Inputs=|++
  base : simulink/Sources/Repeating Sequence Stair  OutValues=f652.PoLC7.l  tsamp=f652.PoLC7.ST  OutMin=[]  OutMax=[]  OutDataTypeStr=double  OutputDataTypeScalingMode=double  OutDataType=fixdt(0,8)  ConRadixGroup=Best Precision: Vector-wise  OutScaling=2^-12
  noise : simulink/Sources/Band-Limited White Noise  Cov=f652.PoLC7.Noise  Ts=f652.PoLC7.NoiseST  seed=f652.PoLC7.NoiseSD
  P : Outport  VectorParamsAs1DForOutWhenUnconnected=off
  wires:
  Sum/1 -> P/1
  noise/1 -> Sum/2
  base/1 -> Sum/1

== system IEEE_13_BUS_Radial/f652/CONTROLLERS/lPoLC8 ==
  Sum : Sum  Inputs=|++
  base : simulink/Sources/Repeating Sequence Stair  OutValues=f652.PoLC8.l  tsamp=f652.PoLC8.ST  OutMin=[]  OutMax=[]  OutDataTypeStr=double  OutputDataTypeScalingMode=double  OutDataType=fixdt(0,8)  ConRadixGroup=Best Precision: Vector-wise  OutScaling=2^-12
  noise : simulink/Sources/Band-Limited White Noise  Cov=f652.PoLC8.Noise  Ts=f652.PoLC8.NoiseST  seed=f652.PoLC8.NoiseSD
  P : Outport  VectorParamsAs1DForOutWhenUnconnected=off
  wires:
  Sum/1 -> P/1
  noise/1 -> Sum/2
  base/1 -> Sum/1

== system IEEE_13_BUS_Radial/f652/CONTROLLERS/lPoLC9 ==
  Sum : Sum  Inputs=|++
  base : simulink/Sources/Repeating Sequence Stair  OutValues=f652.PoLC9.l  tsamp=f652.PoLC9.ST  OutMin=[]  OutMax=[]  OutDataTypeStr=double  OutputDataTypeScalingMode=double  OutDataType=fixdt(0,8)  ConRadixGroup=Best Precision: Vector-wise  OutScaling=2^-12
  noise : simulink/Sources/Band-Limited White Noise  Cov=f652.PoLC9.Noise  Ts=f652.PoLC9.NoiseST  seed=f652.PoLC9.NoiseSD
  P : Outport  VectorParamsAs1DForOutWhenUnconnected=off
  wires:
  Sum/1 -> P/1
  noise/1 -> Sum/2
  base/1 -> Sum/1

== system IEEE_13_BUS_Radial/f652/OPERATIONS GATEWAY/Agent Communications ==
  Enable : EnablePort
  Constant : Constant  Value=0
  Out1 : Outport  VectorParamsAs1DForOutWhenUnconnected=off
  wires:
  Constant/1 -> Out1/1

== system IEEE_13_BUS_Radial/f671/CONTROLLERS/lPoLC1 ==
  Sum : Sum  Inputs=|++
  base : simulink/Sources/Repeating Sequence Stair  OutValues=f671.PoLC1.l  tsamp=f671.PoLC1.ST  OutMin=[]  OutMax=[]  OutDataTypeStr=double  OutputDataTypeScalingMode=double  OutDataType=fixdt(0,8)  ConRadixGroup=Best Precision: Vector-wise  OutScaling=2^-12
  noise : simulink/Sources/Band-Limited White Noise  Cov=f671.PoLC1.Noise  Ts=f671.PoLC1.NoiseST  seed=f671.PoLC1.NoiseSD
  P : Outport  VectorParamsAs1DForOutWhenUnconnected=off
  wires:
  base/1 -> Sum/1
  noise/1 -> Sum/2
  Sum/1 -> P/1

== system IEEE_13_BUS_Radial/f671/CONTROLLERS/lPoLC10 ==
  Sum : Sum  Inputs=|++
  base : simulink/Sources/Repeating Sequence Stair  OutValues=f671.PoLC10.l  tsamp=f671.PoLC10.ST  OutMin=[]  OutMax=[]  OutDataTypeStr=double  OutputDataTypeScalingMode=double  OutDataType=fixdt(0,8)  ConRadixGroup=Best Precision: Vector-wise  OutScaling=2^-12
  noise : simulink/Sources/Band-Limited White Noise  Cov=f671.PoLC10.Noise  Ts=f671.PoLC10.NoiseST  seed=f671.PoLC10.NoiseSD
  P : Outport  VectorParamsAs1DForOutWhenUnconnected=off
  wires:
  base/1 -> Sum/1
  noise/1 -> Sum/2
  Sum/1 -> P/1

== system IEEE_13_BUS_Radial/f671/CONTROLLERS/lPoLC11 ==
  Sum : Sum  Inputs=|++
  base : simulink/Sources/Repeating Sequence Stair  OutValues=f671.PoLC11.l  tsamp=f671.PoLC11.ST  OutMin=[]  OutMax=[]  OutDataTypeStr=double  OutputDataTypeScalingMode=double  OutDataType=fixdt(0,8)  ConRadixGroup=Best Precision: Vector-wise  OutScaling=2^-12
  noise : simulink/Sources/Band-Limited White Noise  Cov=f671.PoLC11.Noise  Ts=f671.PoLC11.NoiseST  seed=f671.PoLC11.NoiseSD
  P : Outport  VectorParamsAs1DForOutWhenUnconnected=off
  wires:
  base/1 -> Sum/1
  noise/1 -> Sum/2
  Sum/1 -> P/1

== system IEEE_13_BUS_Radial/f671/CONTROLLERS/lPoLC12 ==
  Sum : Sum  Inputs=|++
  base : simulink/Sources/Repeating Sequence Stair  OutValues=f671.PoLC12.l  tsamp=f671.PoLC12.ST  OutMin=[]  OutMax=[]  OutDataTypeStr=double  OutputDataTypeScalingMode=double  OutDataType=fixdt(0,8)  ConRadixGroup=Best Precision: Vector-wise  OutScaling=2^-12
  noise : simulink/Sources/Band-Limited White Noise  Cov=f671.PoLC12.Noise  Ts=f671.PoLC12.NoiseST  seed=f671.PoLC12.NoiseSD
  P : Outport  VectorParamsAs1DForOutWhenUnconnected=off
  wires:
  base/1 -> Sum/1
  noise/1 -> Sum/2
  Sum/1 -> P/1

== system IEEE_13_BUS_Radial/f671/CONTROLLERS/lPoLC13 ==
  Sum : Sum  Inputs=|++
  base : simulink/Sources/Repeating Sequence Stair  OutValues=f671.PoLC13.l  tsamp=f671.PoLC13.ST  OutMin=[]  OutMax=[]  OutDataTypeStr=double  OutputDataTypeScalingMode=double  OutDataType=fixdt(0,8)  ConRadixGroup=Best Precision: Vector-wise  OutScaling=2^-12
  noise : simulink/Sources/Band-Limited White Noise  Cov=f671.PoLC13.Noise  Ts=f671.PoLC13.NoiseST  seed=f671.PoLC13.NoiseSD
  P : Outport  VectorParamsAs1DForOutWhenUnconnected=off
  wires:
  base/1 -> Sum/1
  noise/1 -> Sum/2
  Sum/1 -> P/1

== system IEEE_13_BUS_Radial/f671/CONTROLLERS/lPoLC14 ==
  Sum : Sum  Inputs=|++
  base : simulink/Sources/Repeating Sequence Stair  OutValues=f671.PoLC14.l  tsamp=f671.PoLC14.ST  OutMin=[]  OutMax=[]  OutDataTypeStr=double  OutputDataTypeScalingMode=double  OutDataType=fixdt(0,8)  ConRadixGroup=Best Precision: Vector-wise  OutScaling=2^-12
  noise : simulink/Sources/Band-Limited White Noise  Cov=f671.PoLC14.Noise  Ts=f671.PoLC14.NoiseST  seed=f671.PoLC14.NoiseSD
  P : Outport  VectorParamsAs1DForOutWhenUnconnected=off
  wires:
  base/1 -> Sum/1
  noise/1 -> Sum/2
  Sum/1 -> P/1

== system IEEE_13_BUS_Radial/f671/CONTROLLERS/lPoLC15 ==
  Sum : Sum  Inputs=|++
  base : simulink/Sources/Repeating Sequence Stair  OutValues=f671.PoLC15.l  tsamp=f671.PoLC15.ST  OutMin=[]  OutMax=[]  OutDataTypeStr=double  OutputDataTypeScalingMode=double  OutDataType=fixdt(0,8)  ConRadixGroup=Best Precision: Vector-wise  OutScaling=2^-12
  noise : simulink/Sources/Band-Limited White Noise  Cov=f671.PoLC15.Noise  Ts=f671.PoLC15.NoiseST  seed=f671.PoLC15.NoiseSD
  P : Outport  VectorParamsAs1DForOutWhenUnconnected=off
  wires:
  base/1 -> Sum/1
  noise/1 -> Sum/2
  Sum/1 -> P/1

== system IEEE_13_BUS_Radial/f671/CONTROLLERS/lPoLC16 ==
  cv : Inport
  Sum : Sum  Inputs=|++
  Terminator : Terminator
  base : simulink/Sources/Repeating Sequence Stair  OutValues=f671.PoLC16.l  tsamp=f671.PoLC16.ST  OutMin=[]  OutMax=[]  OutDataTypeStr=double  OutputDataTypeScalingMode=double  OutDataType=fixdt(0,8)  ConRadixGroup=Best Precision: Vector-wise  OutScaling=2^-12
  noise : simulink/Sources/Band-Limited White Noise  Cov=f671.PoLC16.Noise  Ts=f671.PoLC16.NoiseST  seed=f671.PoLC16.NoiseSD
  P : Outport  VectorParamsAs1DForOutWhenUnconnected=off
  wires:
  cv/1 -> P/1
  base/1 -> Sum/1
  noise/1 -> Sum/2
  Sum/1 -> Terminator/1

== system IEEE_13_BUS_Radial/f671/CONTROLLERS/lPoLC2 ==
  Sum : Sum  Inputs=|++
  base : simulink/Sources/Repeating Sequence Stair  OutValues=f671.PoLC2.l  tsamp=f671.PoLC2.ST  OutMin=[]  OutMax=[]  OutDataTypeStr=double  OutputDataTypeScalingMode=double  OutDataType=fixdt(0,8)  ConRadixGroup=Best Precision: Vector-wise  OutScaling=2^-12
  noise : simulink/Sources/Band-Limited White Noise  Cov=f671.PoLC2.Noise  Ts=f671.PoLC2.NoiseST  seed=f671.PoLC2.NoiseSD
  P : Outport  VectorParamsAs1DForOutWhenUnconnected=off
  wires:
  base/1 -> Sum/1
  noise/1 -> Sum/2
  Sum/1 -> P/1

== system IEEE_13_BUS_Radial/f671/CONTROLLERS/lPoLC3 ==
  Sum : Sum  Inputs=|++
  base : simulink/Sources/Repeating Sequence Stair  OutValues=f671.PoLC3.l  tsamp=f671.PoLC3.ST  OutMin=[]  OutMax=[]  OutDataTypeStr=double  OutputDataTypeScalingMode=double  OutDataType=fixdt(0,8)  ConRadixGroup=Best Precision: Vector-wise  OutScaling=2^-12
  noise : simulink/Sources/Band-Limited White Noise  Cov=f671.PoLC3.Noise  Ts=f671.PoLC3.NoiseST  seed=f671.PoLC3.NoiseSD
  P : Outport  VectorParamsAs1DForOutWhenUnconnected=off
  wires:
  base/1 -> Sum/1
  noise/1 -> Sum/2
  Sum/1 -> P/1

== system IEEE_13_BUS_Radial/f671/CONTROLLERS/lPoLC4 ==
  Sum : Sum  Inputs=|++
  base : simulink/Sources/Repeating Sequence Stair  OutValues=f671.PoLC4.l  tsamp=f671.PoLC4.ST  OutMin=[]  OutMax=[]  OutDataTypeStr=double  OutputDataTypeScalingMode=double  OutDataType=fixdt(0,8)  ConRadixGroup=Best Precision: Vector-wise  OutScaling=2^-12
  noise : simulink/Sources/Band-Limited White Noise  Cov=f671.PoLC4.Noise  Ts=f671.PoLC4.NoiseST  seed=f671.PoLC4.NoiseSD
  P : Outport  VectorParamsAs1DForOutWhenUnconnected=off
  wires:
  base/1 -> Sum/1
  noise/1 -> Sum/2
  Sum/1 -> P/1

== system IEEE_13_BUS_Radial/f671/CONTROLLERS/lPoLC5 ==
  Sum : Sum  Inputs=|++
  base : simulink/Sources/Repeating Sequence Stair  OutValues=f671.PoLC5.l  tsamp=f671.PoLC5.ST  OutMin=[]  OutMax=[]  OutDataTypeStr=double  OutputDataTypeScalingMode=double  OutDataType=fixdt(0,8)  ConRadixGroup=Best Precision: Vector-wise  OutScaling=2^-12
  noise : simulink/Sources/Band-Limited White Noise  Cov=f671.PoLC5.Noise  Ts=f671.PoLC5.NoiseST  seed=f671.PoLC5.NoiseSD
  P : Outport  VectorParamsAs1DForOutWhenUnconnected=off
  wires:
  base/1 -> Sum/1
  noise/1 -> Sum/2
  Sum/1 -> P/1

== system IEEE_13_BUS_Radial/f671/CONTROLLERS/lPoLC6 ==
  Sum : Sum  Inputs=|++
  base : simulink/Sources/Repeating Sequence Stair  OutValues=f671.PoLC6.l  tsamp=f671.PoLC6.ST  OutMin=[]  OutMax=[]  OutDataTypeStr=double  OutputDataTypeScalingMode=double  OutDataType=fixdt(0,8)  ConRadixGroup=Best Precision: Vector-wise  OutScaling=2^-12
  noise : simulink/Sources/Band-Limited White Noise  Cov=f671.PoLC6.Noise  Ts=f671.PoLC6.NoiseST  seed=f671.PoLC6.NoiseSD
  P : Outport  VectorParamsAs1DForOutWhenUnconnected=off
  wires:
  base/1 -> Sum/1
  noise/1 -> Sum/2
  Sum/1 -> P/1

== system IEEE_13_BUS_Radial/f671/CONTROLLERS/lPoLC7 ==
  Sum : Sum  Inputs=|++
  base : simulink/Sources/Repeating Sequence Stair  OutValues=f671.PoLC7.l  tsamp=f671.PoLC7.ST  OutMin=[]  OutMax=[]  OutDataTypeStr=double  OutputDataTypeScalingMode=double  OutDataType=fixdt(0,8)  ConRadixGroup=Best Precision: Vector-wise  OutScaling=2^-12
  noise : simulink/Sources/Band-Limited White Noise  Cov=f671.PoLC7.Noise  Ts=f671.PoLC7.NoiseST  seed=f671.PoLC7.NoiseSD
  P : Outport  VectorParamsAs1DForOutWhenUnconnected=off
  wires:
  base/1 -> Sum/1
  noise/1 -> Sum/2
  Sum/1 -> P/1

== system IEEE_13_BUS_Radial/f671/CONTROLLERS/lPoLC8 ==
  Sum : Sum  Inputs=|++
  base : simulink/Sources/Repeating Sequence Stair  OutValues=f671.PoLC8.l  tsamp=f671.PoLC8.ST  OutMin=[]  OutMax=[]  OutDataTypeStr=double  OutputDataTypeScalingMode=double  OutDataType=fixdt(0,8)  ConRadixGroup=Best Precision: Vector-wise  OutScaling=2^-12
  noise : simulink/Sources/Band-Limited White Noise  Cov=f671.PoLC8.Noise  Ts=f671.PoLC8.NoiseST  seed=f671.PoLC8.NoiseSD
  P : Outport  VectorParamsAs1DForOutWhenUnconnected=off
  wires:
  base/1 -> Sum/1
  noise/1 -> Sum/2
  Sum/1 -> P/1

== system IEEE_13_BUS_Radial/f671/CONTROLLERS/lPoLC9 ==
  Sum : Sum  Inputs=|++
  base : simulink/Sources/Repeating Sequence Stair  OutValues=f671.PoLC9.l  tsamp=f671.PoLC9.ST  OutMin=[]  OutMax=[]  OutDataTypeStr=double  OutputDataTypeScalingMode=double  OutDataType=fixdt(0,8)  ConRadixGroup=Best Precision: Vector-wise  OutScaling=2^-12
  noise : simulink/Sources/Band-Limited White Noise  Cov=f671.PoLC9.Noise  Ts=f671.PoLC9.NoiseST  seed=f671.PoLC9.NoiseSD
  P : Outport  VectorParamsAs1DForOutWhenUnconnected=off
  wires:
  base/1 -> Sum/1
  noise/1 -> Sum/2
  Sum/1 -> P/1

== system IEEE_13_BUS_Radial/f671/OPERATIONS GATEWAY/Agent Communications ==
  Enable : EnablePort
  Constant : Constant  Value=0
  Out1 : Outport  VectorParamsAs1DForOutWhenUnconnected=off
  wires:
  Constant/1 -> Out1/1

== system IEEE_13_BUS_Radial/f675/CONTROLLERS/lPoLC1 ==
  Sum : Sum  Inputs=|++
  base : simulink/Sources/Repeating Sequence Stair  OutValues=f675.PoLC1.l  tsamp=f675.PoLC1.ST  OutMin=[]  OutMax=[]  OutDataTypeStr=double  OutputDataTypeScalingMode=double  OutDataType=fixdt(0,8)  ConRadixGroup=Best Precision: Vector-wise  OutScaling=2^-12
  noise : simulink/Sources/Band-Limited White Noise  Cov=f675.PoLC1.Noise  Ts=f675.PoLC1.NoiseST  seed=f675.PoLC1.NoiseSD
  P : Outport  VectorParamsAs1DForOutWhenUnconnected=off
  wires:
  Sum/1 -> P/1
  noise/1 -> Sum/2
  base/1 -> Sum/1

== system IEEE_13_BUS_Radial/f675/CONTROLLERS/lPoLC10 ==
  Sum : Sum  Inputs=|++
  base : simulink/Sources/Repeating Sequence Stair  OutValues=f675.PoLC10.l  tsamp=f675.PoLC10.ST  OutMin=[]  OutMax=[]  OutDataTypeStr=double  OutputDataTypeScalingMode=double  OutDataType=fixdt(0,8)  ConRadixGroup=Best Precision: Vector-wise  OutScaling=2^-12
  noise : simulink/Sources/Band-Limited White Noise  Cov=f675.PoLC10.Noise  Ts=f675.PoLC10.NoiseST  seed=f675.PoLC10.NoiseSD
  P : Outport  VectorParamsAs1DForOutWhenUnconnected=off
  wires:
  Sum/1 -> P/1
  noise/1 -> Sum/2
  base/1 -> Sum/1

== system IEEE_13_BUS_Radial/f675/CONTROLLERS/lPoLC11 ==
  Sum : Sum  Inputs=|++
  base : simulink/Sources/Repeating Sequence Stair  OutValues=f675.PoLC11.l  tsamp=f675.PoLC11.ST  OutMin=[]  OutMax=[]  OutDataTypeStr=double  OutputDataTypeScalingMode=double  OutDataType=fixdt(0,8)  ConRadixGroup=Best Precision: Vector-wise  OutScaling=2^-12
  noise : simulink/Sources/Band-Limited White Noise  Cov=f675.PoLC11.Noise  Ts=f675.PoLC11.NoiseST  seed=f675.PoLC11.NoiseSD
  P : Outport  VectorParamsAs1DForOutWhenUnconnected=off
  wires:
  Sum/1 -> P/1
  noise/1 -> Sum/2
  base/1 -> Sum/1

== system IEEE_13_BUS_Radial/f675/CONTROLLERS/lPoLC12 ==
  Sum : Sum  Inputs=|++
  base : simulink/Sources/Repeating Sequence Stair  OutValues=f675.PoLC12.l  tsamp=f675.PoLC12.ST  OutMin=[]  OutMax=[]  OutDataTypeStr=double  OutputDataTypeScalingMode=double  OutDataType=fixdt(0,8)  ConRadixGroup=Best Precision: Vector-wise  OutScaling=2^-12
  noise : simulink/Sources/Band-Limited White Noise  Cov=f675.PoLC12.Noise  Ts=f675.PoLC12.NoiseST  seed=f675.PoLC12.NoiseSD
  P : Outport  VectorParamsAs1DForOutWhenUnconnected=off
  wires:
  Sum/1 -> P/1
  noise/1 -> Sum/2
  base/1 -> Sum/1

== system IEEE_13_BUS_Radial/f675/CONTROLLERS/lPoLC13 ==
  Sum : Sum  Inputs=|++
  base : simulink/Sources/Repeating Sequence Stair  OutValues=f675.PoLC13.l  tsamp=f675.PoLC13.ST  OutMin=[]  OutMax=[]  OutDataTypeStr=double  OutputDataTypeScalingMode=double  OutDataType=fixdt(0,8)  ConRadixGroup=Best Precision: Vector-wise  OutScaling=2^-12
  noise : simulink/Sources/Band-Limited White Noise  Cov=f675.PoLC13.Noise  Ts=f675.PoLC13.NoiseST  seed=f675.PoLC13.NoiseSD
  P : Outport  VectorParamsAs1DForOutWhenUnconnected=off
  wires:
  Sum/1 -> P/1
  noise/1 -> Sum/2
  base/1 -> Sum/1

== system IEEE_13_BUS_Radial/f675/CONTROLLERS/lPoLC14 ==
  Sum : Sum  Inputs=|++
  base : simulink/Sources/Repeating Sequence Stair  OutValues=f675.PoLC14.l  tsamp=f675.PoLC14.ST  OutMin=[]  OutMax=[]  OutDataTypeStr=double  OutputDataTypeScalingMode=double  OutDataType=fixdt(0,8)  ConRadixGroup=Best Precision: Vector-wise  OutScaling=2^-12
  noise : simulink/Sources/Band-Limited White Noise  Cov=f675.PoLC14.Noise  Ts=f675.PoLC14.NoiseST  seed=f675.PoLC14.NoiseSD
  P : Outport  VectorParamsAs1DForOutWhenUnconnected=off
  wires:
  Sum/1 -> P/1
  noise/1 -> Sum/2
  base/1 -> Sum/1

== system IEEE_13_BUS_Radial/f675/CONTROLLERS/lPoLC15 ==
  Sum : Sum  Inputs=|++
  base : simulink/Sources/Repeating Sequence Stair  OutValues=f675.PoLC15.l  tsamp=f675.PoLC15.ST  OutMin=[]  OutMax=[]  OutDataTypeStr=double  OutputDataTypeScalingMode=double  OutDataType=fixdt(0,8)  ConRadixGroup=Best Precision: Vector-wise  OutScaling=2^-12
  noise : simulink/Sources/Band-Limited White Noise  Cov=f675.PoLC15.Noise  Ts=f675.PoLC15.NoiseST  seed=f675.PoLC15.NoiseSD
  P : Outport  VectorParamsAs1DForOutWhenUnconnected=off
  wires:
  Sum/1 -> P/1
  noise/1 -> Sum/2
  base/1 -> Sum/1

== system IEEE_13_BUS_Radial/f675/CONTROLLERS/lPoLC16 ==
  cv : Inport
  Sum : Sum  Inputs=|++
  Terminator : Terminator
  base : simulink/Sources/Repeating Sequence Stair  OutValues=f675.PoLC16.l  tsamp=f675.PoLC16.ST  OutMin=[]  OutMax=[]  OutDataTypeStr=double  OutputDataTypeScalingMode=double  OutDataType=fixdt(0,8)  ConRadixGroup=Best Precision: Vector-wise  OutScaling=2^-12
  noise : simulink/Sources/Band-Limited White Noise  Cov=f675.PoLC16.Noise  Ts=f675.PoLC16.NoiseST  seed=f675.PoLC16.NoiseSD
  P : Outport  VectorParamsAs1DForOutWhenUnconnected=off
  wires:
  Sum/1 -> Terminator/1
  noise/1 -> Sum/2
  base/1 -> Sum/1
  cv/1 -> P/1
